simulink library "cdsWord2Bit"  (Simulink 7.1)
settings Model: Creator=maronsson  LastModifiedBy=maronsson

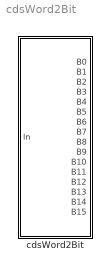
== system cdsWord2Bit ==
  cdsWord2Bit : Subsystem  Tag=cdsWord2Bit  Description=Generate 16 0/1 outputs from single 16-bit integer input
      settings: AttributesFormatString=cdsWord2Bit

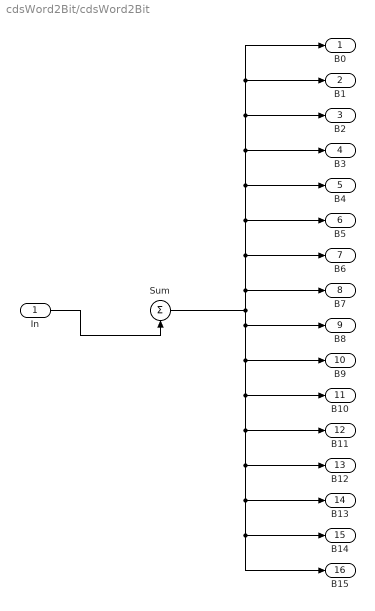
== system cdsWord2Bit/cdsWord2Bit ==
  In : Inport  OutDataType=sfix(16)  OutScaling=2^0
  Sum : Sum  Inputs=|+  OutDataType=sfix(16)  OutScaling=2^0
  B0 : Outport  OutDataType=sfix(16)  OutScaling=2^0
  B1 : Outport  Port=2  OutDataType=sfix(16)  OutScaling=2^0
  B2 : Outport  Port=3  OutDataType=sfix(16)  OutScaling=2^0
  B3 : Outport  Port=4  OutDataType=sfix(16)  OutScaling=2^0
  B4 : Outport  Port=5  OutDataType=sfix(16)  OutScaling=2^0
  B5 : Outport  Port=6  OutDataType=sfix(16)  OutScaling=2^0
  B6 : Outport  Port=7  OutDataType=sfix(16)  OutScaling=2^0
  B7 : Outport  Port=8  OutDataType=sfix(16)  OutScaling=2^0
  B8 : Outport  Port=9  OutDataType=sfix(16)  OutScaling=2^0
  B9 : Outport  Port=10  OutDataType=sfix(16)  OutScaling=2^0
  B10 : Outport  Port=11  OutDataType=sfix(16)  OutScaling=2^0
  B11 : Outport  Port=12  OutDataType=sfix(16)  OutScaling=2^0
  B12 : Outport  Port=13  OutDataType=sfix(16)  OutScaling=2^0
  B13 : Outport  Port=14  OutDataType=sfix(16)  OutScaling=2^0
  B14 : Outport  Port=15  OutDataType=sfix(16)  OutScaling=2^0
  B15 : Outport  Port=16  OutDataType=sfix(16)  OutScaling=2^0
  wires:
  Sum/1 -> B0/1, B1/1, B2/1, B3/1, B4/1, B5/1, B6/1, B7/1, B8/1, B9/1, B10/1, B11/1, B12/1, B13/1, B15/1, B14/1
  In/1 -> Sum/1
